simulink model "tema1_mdl"  (R2019a)
settings: Solver=VariableStepAuto  StartTime=0.0  StopTime=400  RelTol=1e-3
values from neighbouring files (symbols this model uses):
  g = 10    [tema1.m]    (also in tema2.m)
  I = 1.89    [tema1.m]    (also in tema2.m)
  J = 2.77    [tema1.m]    (also in tema2.m)
  k = 0.25    [tema1.m]    (also in tema2.m)
  L = 1.56    [tema1.m]    (also in tema2.m)
  M = 2.82    [tema1.m]    (also in tema2.m)
  zeta = 7.64    [tema1.m]    (also in tema2.m)
settings Model: Creator=cynthia  LastModifiedBy=cynthia

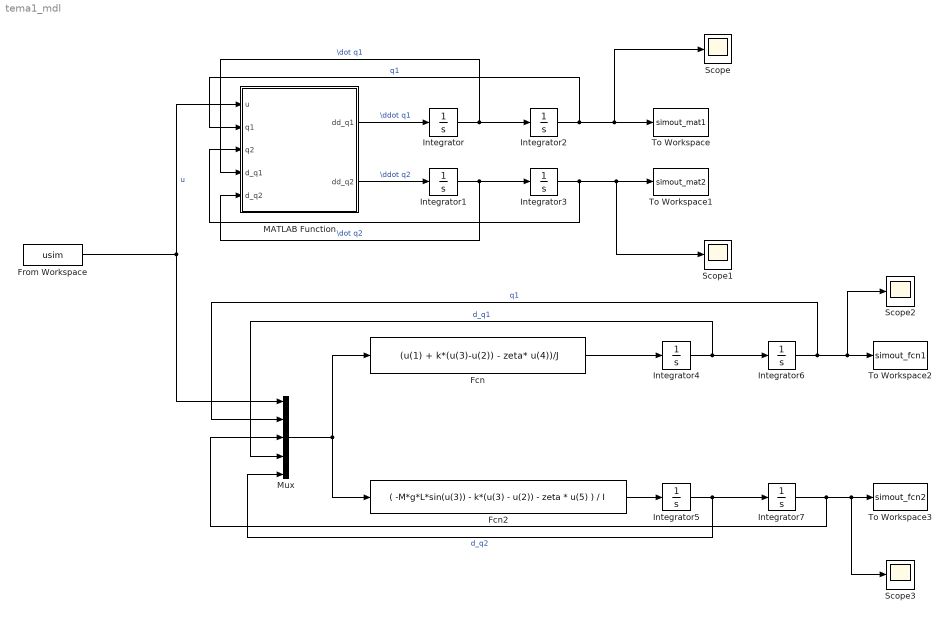
== system tema1_mdl ==
  Fcn : Fcn  Expr=(u(1) + k*(u(3)-u(2)) - zeta* u(4))/J
  Fcn2 : Fcn  Expr=( -M*g*L*sin(u(3)) - k*(u(3) - u(2)) - zeta * u(5) ) / I
  From Workspace : FromWorkspace  VariableName=usim  SampleTime=0
  Integrator{,2,4,6} (4 alike) : Integrator  InitialCondition=1
  Integrator{1,3,5,7} (4 alike) : Integrator
  MATLAB Function : MATLAB Function  TreatAsAtomicUnit=on
  Mux : Mux  Inputs=5
  Scope{,1..3} (4 alike) : Scope
  To Workspace : ToWorkspace  VariableName=simout_mat1  SaveFormat=Timeseries  SampleTime=-1
  To Workspace1 : ToWorkspace  VariableName=simout_mat2  SaveFormat=Timeseries  SampleTime=-1
  To Workspace2 : ToWorkspace  VariableName=simout_fcn1  SaveFormat=Timeseries  SampleTime=-1
  To Workspace3 : ToWorkspace  VariableName=simout_fcn2  SaveFormat=Timeseries  SampleTime=-1
  wires:
  MATLAB Function/1(dd_q1) -> Integrator/1  "\\ddot q1"
  Integrator/1 -> Integrator2/1, MATLAB Function/4(d_q1)  "\\dot q1"
  MATLAB Function/2(dd_q2) -> Integrator1/1  "\\ddot q2"
  Integrator1/1 -> Integrator3/1, MATLAB Function/5(d_q2)  "\\dot q2"
  From Workspace/1 -> MATLAB Function/1(u), Mux/1  "u"
  Integrator2/1 -> Scope/1, To Workspace/1, MATLAB Function/2(q1)  "q1"
  Integrator3/1 -> Scope1/1, To Workspace1/1, MATLAB Function/3(q2)
  Mux/1 -> Fcn/1, Fcn2/1
  Fcn/1 -> Integrator4/1
  Integrator5/1 -> Integrator7/1, Mux/5  "d_q2"
  Integrator4/1 -> Integrator6/1, Mux/4  "d_q1"
  Integrator6/1 -> Scope2/1, To Workspace2/1, Mux/2  "q1"
  Integrator7/1 -> Scope3/1, To Workspace3/1, Mux/3
  Fcn2/1 -> Integrator5/1

== matlab function tema1_mdl/MATLAB Function ==
  data: u input; dd_q1 output; q1 input; q2 input; d_q1 input; d_q2 input; dd_q2 output
function [dd_q1,dd_q2] = fcn(u,q1,q2,d_q1,d_q2)
m = 5.1;
g = 10;
L = 1.56;
zeta = 7.64;
k = 0.25;
J = 2.77; 
I = 1.89;
M = 2.82;

dd_q1 = (u + k*(q2-q1) - zeta*d_q1)/J;
dd_q2 = (-M*g*L*sin(q2) - k*(q2-q1) - zeta*d_q2)/I;


end
